simulink model "amk_real_model"  (R2022b)
settings: Solver=FixedStepAuto  StartTime=0.0  StopTime=0.5  FixedStep=1e-6  RelTol=1e-3
values from neighbouring files (symbols this model uses):
  a_fw = log(9)/trfw    [amk_sim.m]    (also in amk_sim_2.m)
  ac = log(9)/tr    [amk_sim.m]    (also in amk_sim_2.m)
  as = log(9)/trs    [amk_sim.m]    (also in amk_sim_2.m)
  ba = 2*k^2*(as*J - 0)/(np^2*psi)    [amk_sim.m]    (also in amk_sim_2.m = 2*k^2*(as*J - bm)/(np^2*psi))
  bm = 0.02    [amk_sim.m]    (also in amk_sim_2.m = 0.008)
  fsw = 8e3    (= 8000)    [amk_sim.m]    (also in amk_sim_2.m)
  I_base = 85.7    [amk_sim.m]    (also in amk_sim_2.m)
  I_max = 85.7    [amk_sim.m]    (also in amk_sim_2.m)
  Icon = 33.5    [amk_sim.m]    (also in amk_sim_2.m)
  Imax_interval = 1.24    [amk_sim.m]    (also in amk_sim_2.m = 5)
  Ipeak = 85.7    [amk_sim.m]    (also in amk_sim_2.m = 87.5)
  J = 2.5*(2.74e-4)    (= 0.000685)    [amk_sim.m]    (also in amk_sim_2.m = 0.000528)
  k = 1    [amk_sim.m]    (also in amk_sim_2.m)
  ki_s = 2*k^2*as^2*J/(np^2*psi)    [amk_sim.m]    (also in amk_sim_2.m)
  kp_s = 2*k^2*as*J/(np^2*psi)    [amk_sim.m]    (also in amk_sim_2.m)
  Ld = Ldm    (= 0.0004)    [amk_sim.m]    (also in amk_sim_2.m = 0.00012)
  Lq = Lqm    (= 0.00052)    [amk_sim.m]    (also in amk_sim_2.m = 0.00024)
  max_temp = 140    [amk_sim.m]    (also in amk_sim_2.m)
  np = 5    [amk_sim.m]    (also in amk_sim_2.m)
  Peak_power = 45000    [amk_sim.m]    (also in amk_sim_2.m = 50000)
  Peak_regen = -15000    [amk_sim.m]    (also in amk_sim_2.m = -1500000)
  psi = 0.047    [amk_sim.m]    (also in amk_sim_2.m = 0.05077789)
  rpm_nom = 20000    [amk_sim.m]    (also in amk_sim_2.m = 12000)
  Rs = 202.5e-3    (= 0.2025)    [amk_sim.m]    (also in amk_sim_2.m)
  sample_time = 1e-4    (= 0.0001)    [amk_sim.m]    (also in amk_sim_2.m = 1e-06)
  temp_threshold = 100    [amk_sim.m]    (also in amk_sim_2.m)
  u_dc = 550    [amk_sim.m]    (also in amk_sim_2.m)
  u_nom = u_dc*k    (= 550)    [amk_sim.m]    (also in amk_sim_2.m)
undefined symbols (not defined in the file or in its folder): Icutoff, rc1, rc2, rc3, rc4, rc5
libraries: spsIGBTDiodeLib x6, simulink x5, spsCurrentMeasurementLib x3, spsSeriesRLCBranchLib x3, spsDCVoltageSourceLib x1, spsPermanentMagnetSynchronousMachineLib x1, dspstat3 x1, spsThreePhaseVIMeasurementLib x1, spsMultimeterLib x1, spsTriangleGeneratorLib x1, sps_lib x1
(part 1 of 4)
settings Model: Creator=alexa  LastModifiedBy=alexa

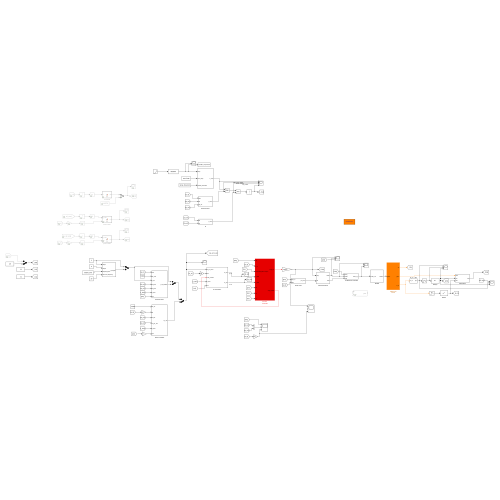
[thumbnail: Simulink's stored preview of the top-level diagram]
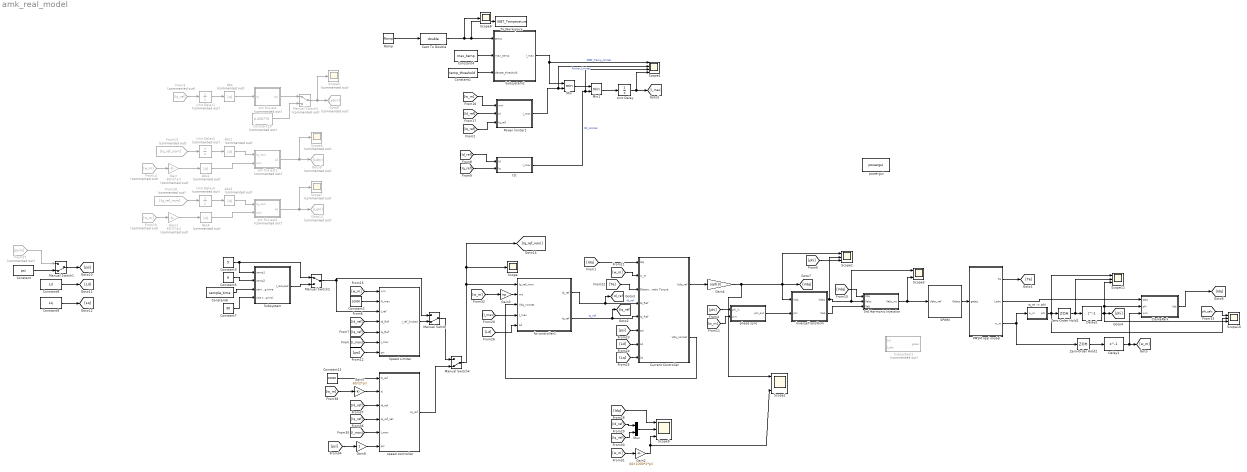
== system amk_real_model ==
  3rd Harmonic Injection : Subsystem
  Abs{,1..4} (5 alike) : Abs  Commented=on  SaturateOnIntegerOverflow=off
  Cast To Double : DataTypeConversion  OutDataTypeStr=double  SaturateOnIntegerOverflow=off  RndMeth=Floor
  ClarkePark : Subsystem
  Constant : Constant  Value=psi
  Constant1 : Constant  Value=temp_threshold
  Constant10 : Constant  Commented=on  Value=0.050779
  Constant11 : Constant  Value=15000
  Constant2 : Constant  Value=10000
  Constant3 : Constant  Value=5
  Constant4 : Constant  Value=max_temp
  Constant5 : Constant  Value=9
  Constant6 : Constant  Value=sample_time
  Constant7 : Constant  Value=30
  Constant8 : Constant  Value=Ld
  Constant9 : Constant  Value=Lq
  Current Controller : Subsystem
  Delay1 : Delay  DelayLength=1  InitialCondition=0  UseCircularBuffer=on
  Delay2 : Delay  DelayLength=1  InitialCondition=0  UseCircularBuffer=on
  From13 : From  Commented=on  GotoTag=Iq_ref_nom
  From14 : From  Commented=on  GotoTag=w_m
  From18 : From  Commented=on  GotoTag=Iq_ref_nom
  From19 : From  Commented=on  GotoTag=w_m
  From27 : From  Commented=on  GotoTag=psim
  From3 : From  Commented=on  GotoTag=Iq_ref
  Gain : Gain  Commented=on  Gain=60/(2*pi)
  Gain1 : Gain  Commented=on  Gain=60/(2*pi)
  Gain2 : Gain  Gain=60/(1000*2*pi)
  Gain3 : Gain  Gain=np
  Gain4 : Gain  Gain=sqrt(3)
  Gain5 : Gain  Gain=60/(2*pi)
  Gain6 : Gain
  Goto13 : Goto  Commented=on  GotoTag=Lqm
  Goto8 : Goto  Commented=on  GotoTag=psim
  Goto9 : Goto  Commented=on  GotoTag=Ldm
  I2t : Subsystem
  InverseTransform : Subsystem
  Manual Switch : ManualSwitch  CurrentSetting=0
  Manual Switch1 : ManualSwitch  CurrentSetting=0
  Manual Switch2 : ManualSwitch
  Manual Switch3 : ManualSwitch  Commented=on
  Manual Switch4 : ManualSwitch  CurrentSetting=0
  Min : MinMax  Inputs=2
  Min1 : MinMax  Inputs=2
  Mux : Mux  Inputs=2
  PMSM real model : Subsystem
  Power limiter1 : Subsystem
  Ramp : simulink/Sources/Ramp  slope=1  start=0  InitialOutput=30
  SPWM : Subsystem
  Scope : Scope
  Scope{1..3,9..11} (6 alike) : Scope  NumInputPorts=3
  Scope4 : Scope  NumInputPorts=4
  Scope5 : Scope  Commented=on
  Scope6 : Scope  Commented=on
  Scope7 : Scope  Commented=on
  Scope8 : Scope
  Speed Limiter : Subsystem
  Subsystem : Subsystem
  Subsystem1 : Subsystem  Commented=on
  Subsystem2 : Subsystem
  To Workspace : ToWorkspace  VariableName=IGBT_Temperature  SampleTime=-1
  Unit Delay : UnitDelay  SampleTime=-1  HasFrameUpgradeWarning=on
  Unit Delay1 : UnitDelay  Commented=on  SampleTime=-1  HasFrameUpgradeWarning=on
  Unit Delay2 : UnitDelay  Commented=on  SampleTime=-1  HasFrameUpgradeWarning=on
  Unit Delay3 : UnitDelay  Commented=on  SampleTime=-1  HasFrameUpgradeWarning=on
  Zero-Order Hold1 : ZeroOrderHold  SampleTime=62e-6
  Zero-Order Hold2 : ZeroOrderHold  SampleTime=62e-6
  fw controller1 : Subsystem
  phase sync : Subsystem
  pm flux est : MATLAB Function  Commented=on  TreatAsAtomicUnit=on
  pm flux est1 : MATLAB Function  Commented=on  TreatAsAtomicUnit=on
  pm flux est2 : MATLAB Function  Commented=on  TreatAsAtomicUnit=on
  powergui : sps_lib/powergui  Priority=1  SimulationMode=Continuous  SampleTime=50e-6  frequency=60  Iterations=50  frequencyindice=0  Pbase=100e6  ErrMax=1e-4  UnitsV=kV  UnitsW=MW  buscounter=0  FunctionMessages=off  echomessages=off  EnableUseOfTLC=off  CurrentSourceSwitches=off  DisableSnubberDevices=off  DisableRonSwitches=off  DisableVfSwitches=off  DisplayEquations=off  AutomaticDiscreteSolvers=off  SolverType=Tustin/Backward Euler (TBE)  Interpol=off  ExternalGateDelay=off  methode=off  Ts=100  x0status=blocks  SPID=on  SwTol=0  HookPort=off  NonlinearTolerance=0  nMaxIteration=15  ContinueOnMaxIteration=off  RestoreLinks=warning  ResistiveCurrentMeasurement=off  Frange=[0:2:500]  Ylog=off  Xlog=on  ShowGrid=off  save=off  variable=ZData  structure=0  ZoomFFT=off  StartTime=0.0  cycles=1  DisplayStyle=1  fundamental=60  FreqAxis=off  MaxFrequency=1000  frequencyindicesteady=1  RmsSteady=1  display=off
  speed controller : Subsystem
  "w_m -> phi" : Subsystem
  wires:
  3rd Harmonic Injection/1(Vabc_inj) -> SPWM/1(Uabc_ref), Scope3/3
  Zero-Order Hold1/1 -> Scope11/2, Delay2/1
  InverseTransform/2(Vab) -> 3rd Harmonic Injection/3(Vab)
  [w_m] -> phase sync/2(wm)
  "w_m -> phi"/1(phi) -> Scope10/2, Scope11/1, Zero-Order Hold1/1
  [phi] -> phase sync/1(phi_in)
  phase sync/1(phi_out) -> InverseTransform/2(phi)
  [Vdq] -> 3rd Harmonic Injection/1(Vdq)
  [phi] -> Scope1/3
  InverseTransform/1(Vabc) -> Scope1/2, Scope3/1, 3rd Harmonic Injection/2(Vabc)
  ClarkePark/1(Idq) -> [Idq]
  PMSM real model/2(I_abc) -> ClarkePark/1(Iabc)
  PMSM real model/3(w_m) -> "w_m -> phi"/1(w_m), Zero-Order Hold2/1
  SPWM/1(Gates) -> PMSM real model/1("gates ")
  PMSM real model/1(Te) -> [Te]
  Current Controller/1("Udq_ref ") -> Gain4/1
  [Iq_ref] -> Mux/2
  From27/1 -> Manual Switch1/1
  [w_m] -> Gain2/1
  From3/1 -> Unit Delay1/1
  Constant10/1 -> Manual Switch3/2
  Abs/1 -> pm flux est/1(Iq)
  Gain/1 -> Abs2/1
  Subsystem/1(I_ramped) -> Manual Switch2/2
  Manual Switch2/1 -> Speed Limiter/3(I_ref), Manual Switch/1
  pm flux est/1(psi) -> Manual Switch3/1
  [Idq] -> Scope9/1
  Abs2/1 -> pm flux est1/2(rpm)
  Constant/1 -> Manual Switch1/2
  [Ld] -> Current Controller/7(Ld)
  pm flux est1/1(Ld) -> Goto9/1, Scope6/1
  Abs1/1 -> pm flux est1/1(Iq_nom)
  Unit Delay2/1 -> Abs1/1
  From13/1 -> Unit Delay2/1
  Constant9/1 -> [Lq]
  [Id_ref] -> Mux/1
  pm flux est2/1(Lq) -> Scope7/1, Goto13/1
  [psi] -> Current Controller/6(psi)
  Gain2/1 -> Scope9/3, Scope2/3
  [Lq] -> Current Controller/8(Lq)
  Manual Switch3/1 -> Scope5/1, Goto8/1
  From14/1 -> Gain/1
  Abs3/1 -> pm flux est2/1(Iq_nom)
  [Id_ref] -> Speed Limiter/4(Id_Ref)
  [Iq_ref] -> Speed Limiter/5(Iq_Ref)
  Mux/1 -> Scope9/2
  From18/1 -> Unit Delay3/1
  Power limiter1/1(I_max) -> Scope4/2, Min/2  "Power_Limiter"
  Constant7/1 -> Subsystem/4(rise time (Amp/ms))
  [psi] -> Speed Limiter/7(psi)
  [Iq_ref] -> Power limiter1/3(Iq_ref)
  [w_m] -> Power limiter1/1(wm)
  Constant1/1 -> Subsystem2/3(derate_threshold)
  Unit Delay/1 -> Scope4/4, [I_max]
  [w_m] -> Gain3/1
  Unit Delay1/1 -> Abs/1
  Gain1/1 -> Abs4/1
  fw controller1/1(Id_ref) -> Current Controller/4(Id_Ref), [Id_ref]  "Id_ref"
  I2t/1(I_max) -> Scope4/3, Min1/2  "I2t_Limiter"
  Abs4/1 -> pm flux est2/2(rpm)
  Subsystem2/1(I_max) -> Min/1, Scope4/1  "IGBT_Temp_limiter"
  Speed Limiter/1(I_ref_limited) -> Manual Switch/2
  [I_max] -> Speed Limiter/6(I_max)
  Unit Delay3/1 -> Abs3/1
  [Iq_ref] -> I2t/2(Iq)
  From19/1 -> Gain1/1
  Constant5/1 -> Subsystem/2(ramp2)
  fw controller1/2(Iq_ref) -> [Iq_ref], Current Controller/5(Iq_Ref)  "Iq_ref"
  [I_max] -> fw controller1/4(I_max)
  Constant4/1 -> Subsystem2/2(max_temp)
  Constant6/1 -> Subsystem/3(sampling time)
  Min/1 -> Min1/1
  [w_m] -> Current Controller/2(w_m)
  [Ld] -> fw controller1/5(Ld)
  [Id_ref] -> I2t/1(Id)
  Constant3/1 -> Subsystem/1(ramp1), Manual Switch2/1
  Current Controller/2(Vdq_nonsat) -> fw controller1/3(Vdq_nonsat)
  Gain3/1 -> fw controller1/2(we)
  [Te] -> Current Controller/3(Electromagnetic Torque)
  Constant2/1 -> Speed Limiter/2(N_max)
  [w_m] -> Speed Limiter/1(wm)
  Cast To Double/1 -> Subsystem2/1(temp), To Workspace/1, Scope8/1
  Min1/1 -> Unit Delay/1
  Ramp/1 -> Cast To Double/1
  [Id_ref] -> Power limiter1/2(Id)
  Manual Switch1/1 -> [psi]
  Constant8/1 -> [Ld]
  [Idq] -> Current Controller/1(Idq)
  Gain4/1 -> Scope2/1, InverseTransform/1(Vdq), Scope1/1, [Vdq]
  Zero-Order Hold2/1 -> Delay1/1
  Delay1/1 -> [w_m], ClarkePark/3(wm)
  Delay2/1 -> Scope11/3, ClarkePark/2(phi), Scope10/3, [phi]
  [phi_calc] -> Scope10/1
  speed controller/1(Iq_ref) -> Manual Switch4/2
  Manual Switch/1 -> Manual Switch4/1
  Manual Switch4/1 -> fw controller1/1(Iq_ref_nom), Scope/1, [Iq_ref_nom]
  [psi] -> Gain6/1
  [I_max] -> speed controller/5(I_max)
  [Iq_ref] -> speed controller/4(Iq_ref_sat)
  [Id_ref] -> speed controller/3(Id_ref)
  Gain5/1 -> speed controller/2(N)
  [w_m] -> Gain5/1
  Constant11/1 -> speed controller/1(N_ref)
  Gain6/1 -> speed controller/6(psi)

== system amk_real_model/3rd Harmonic Injection ==
  note: 3rd harmonic
  Vdq : Inport
  Vabc : Inport  Port=2
  Vab : Inport  Port=3
  Atan2 : Trigonometry  Operator=atan2
  Demux : Demux  Outputs=2
  Demux1 : Demux  Outputs=2
  Gain : Gain  Gain=3
  Gain1 : Gain  Gain=2/sqrt(3)
  Gain2 : Gain  Gain=2/(sqrt(3)*6)
  Product : Product
  Sin : Trigonometry
  Sqrt : Sqrt
  Square : Math  Operator=square
  Square1 : Math  Operator=square
  Sum : Sum  Inputs=|++
  Sum1 : Sum  Inputs=|++
  Vabc_inj : Outport
  wires:
  Vdq/1 -> Demux/1
  Demux/1 -> Square/1
  Demux/2 -> Square1/1
  Square/1 -> Sum/1
  Square1/1 -> Sum/2
  Sum/1 -> Sqrt/1
  Vab/1 -> Demux1/1
  Demux1/1 -> Atan2/1
  Demux1/2 -> Atan2/2
  Atan2/1 -> Gain/1
  Gain/1 -> Sin/1
  Sqrt/1 -> Product/1
  Sin/1 -> Product/2
  Vabc/1 -> Gain1/1
  Product/1 -> Gain2/1
  Gain2/1 -> [mod_3rd]
  Gain1/1 -> Sum1/1
  [mod_3rd] -> Sum1/2
  Sum1/1 -> Vabc_inj/1

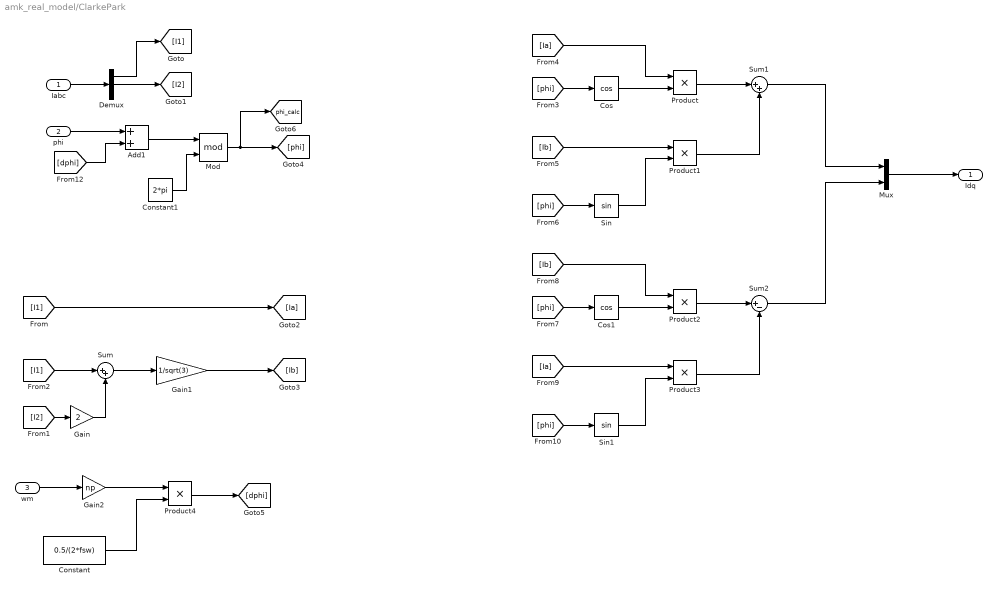
== system amk_real_model/ClarkePark ==
  Iabc : Inport
  phi : Inport  Port=2
  wm : Inport  Port=3
  Add1 : Sum
  Constant : Constant  Value=0.5/(2*fsw)
  Constant1 : Constant  Value=2*pi
  Cos : Trigonometry  Operator=cos
  Cos1 : Trigonometry  Operator=cos
  Demux : Demux  Outputs=3
  Gain : Gain  Gain=2
  Gain1 : Gain  Gain=1/sqrt(3)
  Gain2 : Gain  Gain=np
  Mod : Math  Operator=mod
  Mux : Mux  Inputs=2
  Product{,1..4} (5 alike) : Product
  Sin : Trigonometry
  Sin1 : Trigonometry
  Sum : Sum  Inputs=|++
  Sum1 : Sum  Inputs=|++
  Sum2 : Sum  Inputs=|+-
  Idq : Outport
  tag scope: phi_calc=global
  wires:
  Iabc/1 -> Demux/1
  Demux/1 -> [I1]
  Demux/2 -> [I2]
  [I1] -> [Ia]
  [I1] -> Sum/1
  [I2] -> Gain/1
  Gain/1 -> Sum/2
  Sum/1 -> Gain1/1
  Gain1/1 -> [Ib]
  Cos/1 -> Product/2
  [Ia] -> Product/1
  Product/1 -> Sum1/1
  [phi] -> Sin/1
  [Ib] -> Product1/1
  Sin/1 -> Product1/2
  Product1/1 -> Sum1/2
  Sum1/1 -> Mux/1
  Mux/1 -> Idq/1
  Product3/1 -> Sum2/2
  Sin1/1 -> Product3/2
  [Ia] -> Product3/1
  [phi] -> Sin1/1
  Product2/1 -> Sum2/1
  [Ib] -> Product2/1
  Cos1/1 -> Product2/2
  [phi] -> Cos1/1
  Sum2/1 -> Mux/2
  wm/1 -> Gain2/1
  Gain2/1 -> Product4/1
  Constant/1 -> Product4/2
  Product4/1 -> [dphi]
  [phi] -> Cos/1
  [dphi] -> Add1/2
  phi/1 -> Add1/1
  Add1/1 -> Mod/1
  Mod/1 -> [phi_calc], [phi]
  Constant1/1 -> Mod/2

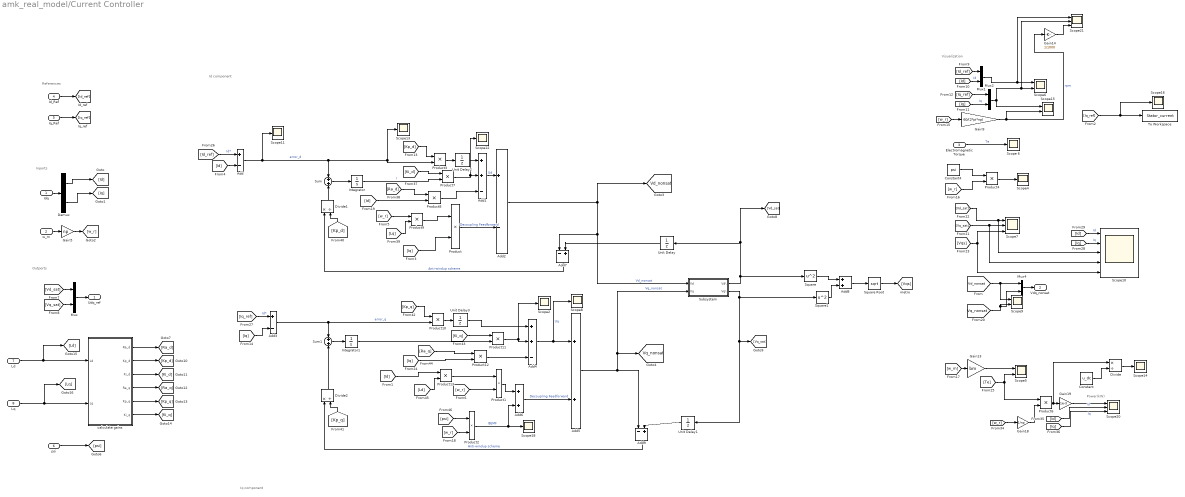
== system amk_real_model/Current Controller ==
  note: References
  note: Id component
  note: Iq component
  note: Inports
  note: Outports
  note: Visualization
  note: Power(kW)
  Idq : Inport
  w_m : Inport  Port=2
  Electromagnetic Torque : Inport  Port=3
  Id_Ref : Inport  Port=4
  Iq_Ref : Inport  Port=5
  psi : Inport  Port=6
  Ld : Inport  Port=7
  Lq : Inport  Port=8
  Add : Sum  Inputs=+-
  Add1 : Sum  Inputs=++-
  Add2 : Sum  Inputs=+-
  Add3 : Sum  Inputs=+-
  Add4 : Sum  Inputs=++-
  Add5 : Sum
  Add6 : Sum
  Add7 : Sum  Inputs=-+
  Add8 : Sum
  Add9 : Sum  Inputs=-+
  Constant : Constant  Value=u_dc
  Constant4 : Constant  Value=psi
  Demux : Demux  Outputs=2
  Divide : Product  Inputs=*/
  Divide1 : Product  Inputs=*/
  Divide2 : Product  Inputs=*/
  Gain13 : Gain  Gain=bm
  Gain14 : Gain  Gain=1/1000
  Gain18 : Gain  Gain=1/np
  Gain19 : Gain  Gain=1e-3
  Gain5 : Gain  Gain=np
  Gain9 : Gain  Gain=60/(2*pi*np)
  Integrator : Integrator
  Integrator1 : Integrator
  Mux{,1..2,4} (4 alike) : Mux  Inputs=2
  Product{,1..4,6..13} (13 alike) : Product
  Scope 6 : Scope
  Scope10 : Scope  NumInputPorts=5
  Scope{2,4,8,11..14,16,18} (9 alike) : Scope
  Scope{5..6,9,15} (4 alike) : Scope  NumInputPorts=2
  Scope20 : Scope  NumInputPorts=3
  Scope21 : Scope  NumInputPorts=3
  Scope7 : Scope  NumInputPorts=3
  Square : Math  Operator=square
  Square Root : Sqrt
  Square1 : Math  Operator=square
  Subsystem : Subsystem
  Sum : Sum
  Sum1 : Sum
  To Workspace : ToWorkspace  VariableName=Stator_current  SampleTime=-1
  Unit Delay{,1..3} (4 alike) : UnitDelay  SampleTime=-1  HasFrameUpgradeWarning=on
  calculate gains : Subsystem
  "Udq_ref " : Outport  VectorParamsAs1DForOutWhenUnconnected=off
  Vdq_nonsat : Outport  Port=2
  tag scope: Vd_nonsat=global, Vq_nonsat=global
  wires:
  Product11/1 -> Add4/2, Scope2/1
  Add4/1 -> Scope8/1, Add5/1  "Uq"
  Add1/1 -> Add2/1  "Ud"
  Product9/1 -> Product/1
  Product10/1 -> Unit Delay3/1
  Sum/1 -> Integrator/1
  Product3/1 -> Unit Delay2/1
  [w_r] -> Product1/2
  Product13/1 -> Product1/1
  Idq/1 -> Demux/1
  Product/1 -> Add2/2  "Decoupling Feedforward"
  Divide1/1 -> Sum/2
  Add2/1 -> [Vd_nonsat], Subsystem/1(Vd), Add7/1  "Vd_nonsat"
  Add7/1 -> Divide1/1  "Anti-windup scheme"
  Sum1/1 -> Integrator1/1
  Add5/1 -> Add9/1, Subsystem/2(Vq), [Vq_nonsat]  "Vq_nonsat"
  Divide2/1 -> Sum1/2
  Add9/1 -> Divide2/1  "Anti-windup scheme"
  Demux/1 -> [Id]
  Demux/2 -> [Iq]
  w_m/1 -> Gain5/1
  Gain5/1 -> [w_r]
  [Vd_sat] -> Mux/1
  [Vq_sat] -> Mux/2
  Mux/1 -> "Udq_ref "/1
  [Id] -> Add/2
  Mux1/1 -> Scope21/1, Scope6/1
  [Id_ref] -> Mux1/1
  [Id] -> Mux1/2  "Id"
  [Iq_ref] -> Mux2/1
  [Iq] -> Mux2/2  "Iq"
  [w_r] -> Gain9/1
  Gain9/1 -> Scope15/2, Gain14/1  "rpm"
  [psi] -> Product2/1
  Product1/1 -> Add6/1
  Add6/1 -> Add5/2  "Decoupling Feedforward"
  Add/1 -> Product3/2, Scope13/1, Sum/1, Scope11/1  "error_d"
  Add3/1 -> Product10/2, Sum1/1  "error_q"
  [Iq] -> Add3/2
  Product7/1 -> Scope12/1, Add1/2
  Square1/1 -> Add8/2
  Square/1 -> Add8/1
  Add8/1 -> Square Root/1
  [Vd_nonsat] -> Scope9/1, Mux4/1
  [Vq_nonsat] -> Mux4/2, Scope9/2
  Square Root/1 -> [Vqs]
  [Vd_sat] -> Scope10/3, Scope7/1
  [Vq_sat] -> Scope10/4, Scope7/2
  [Vqs] -> Scope7/3, Scope10/5
  [w_r] -> Product4/2
  Constant4/1 -> Product4/1
  Product4/1 -> Scope4/1
  Id_Ref/1 -> [Id_ref]
  Iq_Ref/1 -> [Iq_ref]
  Gain13/1 -> Scope5/1
  [Te] -> Product6/1, Scope5/2
  [w_m] -> Gain13/1
  Mux2/1 -> Scope21/2, Scope6/2, Scope15/1
  [Iq] -> Scope10/2  "Iq"
  [Id] -> Scope10/1  "Id"
  [Id_ref] -> Add/1  "Id*"
  Subsystem/1(Vd\) -> Square/1, [Vd_sat], Unit Delay/1
  Subsystem/2(Vq\) -> Square1/1, [Vq_sat], Unit Delay1/1
  [w_r] -> Product2/2
  Product2/1 -> Scope18/1, Add6/2  "BEMF"
  Mux4/1 -> Vdq_nonsat/1
  [Iq_ref] -> Add3/1  "Id*"
  Gain19/1 -> Scope20/1
  [Iq] -> Scope20/3  "Iq"
  [Id] -> Scope20/2  "Id"
  Gain18/1 -> Product6/2
  Product6/1 -> Divide/1, Gain19/1
  [w_r] -> Gain18/1
  Product12/1 -> Add4/3
  Product8/1 -> Add1/3
  Constant/1 -> Divide/2
  Divide/1 -> Scope14/1
  [Id] -> Product8/2
  [Iq] -> Product/2
  [Iq_ref] -> To Workspace/1, Scope16/1
  Electromagnetic Torque/1 -> Scope 6/1  "Te"
  Unit Delay/1 -> Add7/2
  Unit Delay1/1 -> Add9/2
  Gain14/1 -> Scope21/3
  [Kp_d] -> Product3/1
  Integrator/1 -> Product7/2  "I"
  [Ki_d] -> Product7/1
  [Ra_d] -> Product8/1
  [w_r] -> Product9/1
  [Lq] -> Product9/2
  [Kp_d] -> Divide1/2
  [Kp_q] -> Divide2/2
  [Kp_q] -> Product10/1
  [Ki_q] -> Product11/1
  Integrator1/1 -> Product11/2
  [Iq] -> Product12/2
  [Ra_q] -> Product12/1
  [Ld] -> Product13/2
  [Id] -> Product13/1
  Ld/1 -> [Ld], calculate gains/1(Ld)
  Lq/1 -> [Lq], calculate gains/2(Lq)
  psi/1 -> [psi]
  calculate gains/1(Ra_d) -> [Ra_d]
  calculate gains/2(Kp_d) -> [Kp_d]
  calculate gains/3(Ki_d) -> [Ki_d]
  calculate gains/4(Ra_q) -> [Ra_q]
  calculate gains/5(Kp_q) -> [Kp_q]
  calculate gains/6(Ki_q) -> [Ki_q]
  Unit Delay2/1 -> Add1/1
  Unit Delay3/1 -> Add4/1

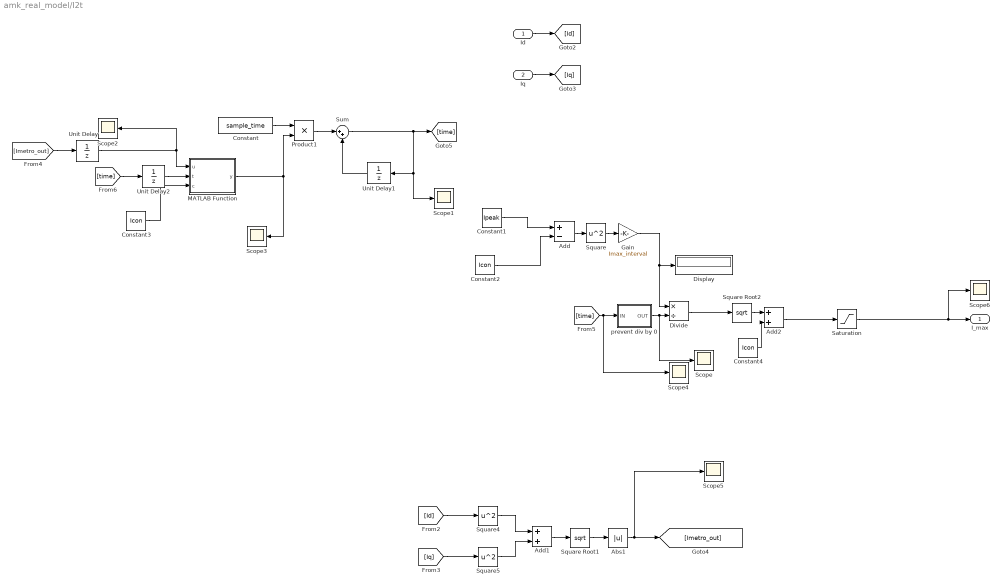
== system amk_real_model/I2t ==
  Id : Inport
  Iq : Inport  Port=2
  Abs1 : Abs  SaturateOnIntegerOverflow=off
  Add : Sum  Inputs=+-
  Add1 : Sum
  Add2 : Sum
  Constant : Constant  Value=sample_time
  Constant1 : Constant  Value=Ipeak
  Constant2 : Constant  Value=Icon
  Constant3 : Constant  Value=Icon
  Constant4 : Constant  Value=Icon
  Display : Display
  Divide : Product  Inputs=*/
  Gain : Gain  Gain=Imax_interval
  MATLAB Function : MATLAB Function  TreatAsAtomicUnit=on
  Product1 : Product
  Saturation : Saturate  UpperLimit=I_max  LowerLimit=0
  Scope{,1..6} (7 alike) : Scope
  Square : Math  Operator=square
  Square Root1 : Sqrt
  Square Root2 : Sqrt
  Square4 : Math  Operator=square
  Square5 : Math  Operator=square
  Sum : Sum  Inputs=|++
  Unit Delay : UnitDelay  SampleTime=-1  HasFrameUpgradeWarning=on
  Unit Delay1 : UnitDelay  SampleTime=-1  HasFrameUpgradeWarning=on
  Unit Delay2 : UnitDelay  SampleTime=-1  HasFrameUpgradeWarning=on
  prevent div by 0 : Subsystem
  I_max : Outport
  wires:
  Iq/1 -> [Iq]
  Id/1 -> [Id]
  Divide/1 -> Square Root2/1
  prevent div by 0/1(OUT) -> Scope/1, Divide/2
  [time] -> Scope4/1, prevent div by 0/1(IN)
  Sum/1 -> Unit Delay1/1, Scope1/1, [time]
  [Imetro_out] -> Unit Delay/1
  [time] -> Unit Delay2/1
  Unit Delay1/1 -> Sum/2
  Add1/1 -> Square Root1/1
  Square5/1 -> Add1/2
  Square4/1 -> Add1/1
  Square Root1/1 -> Abs1/1
  Constant/1 -> Product1/1
  Product1/1 -> Sum/1
  MATLAB Function/1(y) -> Product1/2, Scope3/1
  Constant3/1 -> MATLAB Function/3(c)
  Abs1/1 -> Scope5/1, [Imetro_out]
  Saturation/1 -> I_max/1, Scope6/1
  Unit Delay/1 -> MATLAB Function/1(u), Scope2/1
  Unit Delay2/1 -> MATLAB Function/2(t)
  Gain/1 -> Display/1, Divide/1
  Constant1/1 -> Add/1
  Add/1 -> Square/1
  Constant2/1 -> Add/2
  Square Root2/1 -> Add2/1
  Add2/1 -> Saturation/1
  Constant4/1 -> Add2/2
  Square/1 -> Gain/1
  [Id] -> Square4/1
  [Iq] -> Square5/1

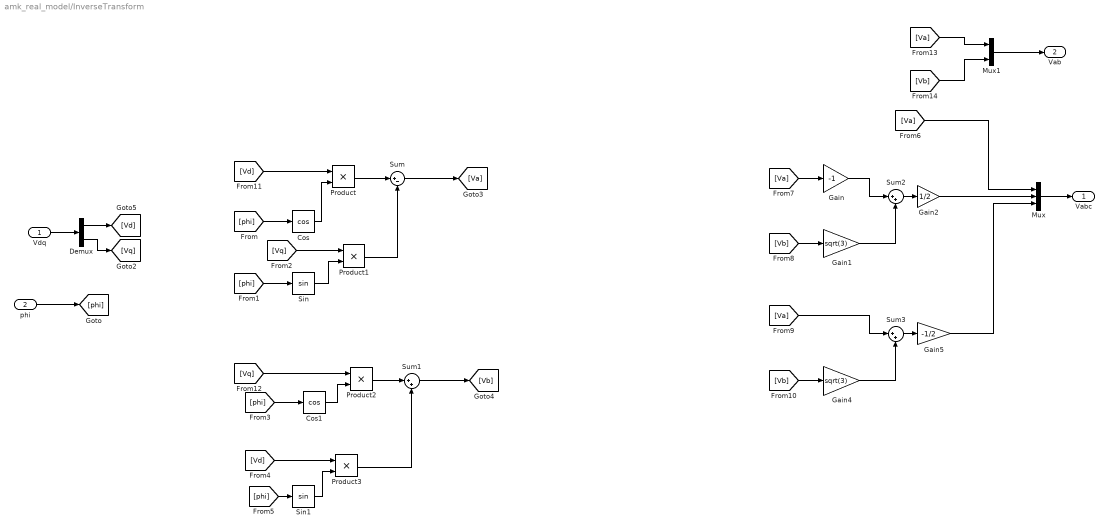
== system amk_real_model/InverseTransform ==
  Vdq : Inport
  phi : Inport  Port=2
  Cos : Trigonometry  Operator=cos
  Cos1 : Trigonometry  Operator=cos
  Demux : Demux  Outputs=2
  Gain : Gain  Gain=-1
  Gain1 : Gain  Gain=sqrt(3)
  Gain2 : Gain  Gain=1/2
  Gain4 : Gain  Gain=sqrt(3)
  Gain5 : Gain  Gain=-1/2
  Mux : Mux  Inputs=3
  Mux1 : Mux  Inputs=2
  Product{,1..3} (4 alike) : Product
  Sin : Trigonometry
  Sin1 : Trigonometry
  Sum : Sum  Inputs=|+-
  Sum1 : Sum  Inputs=|++
  Sum2 : Sum  Inputs=|++
  Sum3 : Sum  Inputs=|++
  Vabc : Outport
  Vab : Outport  Port=2
  wires:
  phi/1 -> [phi]
  [phi] -> Cos/1
  Cos/1 -> Product/2
  Product/1 -> Sum/1
  [phi] -> Sin/1
  [Vq] -> Product1/1
  Sin/1 -> Product1/2
  Product1/1 -> Sum/2
  Cos1/1 -> Product2/2
  [phi] -> Cos1/1
  Product2/1 -> Sum1/1
  Sin1/1 -> Product3/2
  [phi] -> Sin1/1
  [Vd] -> Product3/1
  Product3/1 -> Sum1/2
  Sum/1 -> [Va]
  Sum1/1 -> [Vb]
  [Va] -> Mux/1
  [Va] -> Gain/1
  [Vb] -> Gain1/1
  Gain/1 -> Sum2/1
  Gain1/1 -> Sum2/2
  Sum2/1 -> Gain2/1
  Gain2/1 -> Mux/2
  Sum3/1 -> Gain5/1
  Gain4/1 -> Sum3/2
  [Va] -> Sum3/1
  [Vb] -> Gain4/1
  Vdq/1 -> Demux/1
  Demux/1 -> [Vd]
  Demux/2 -> [Vq]
  [Vd] -> Product/1
  [Vq] -> Product2/1
  Gain5/1 -> Mux/3
  Mux/1 -> Vabc/1
  Mux1/1 -> Vab/1
  [Va] -> Mux1/1
  [Vb] -> Mux1/2

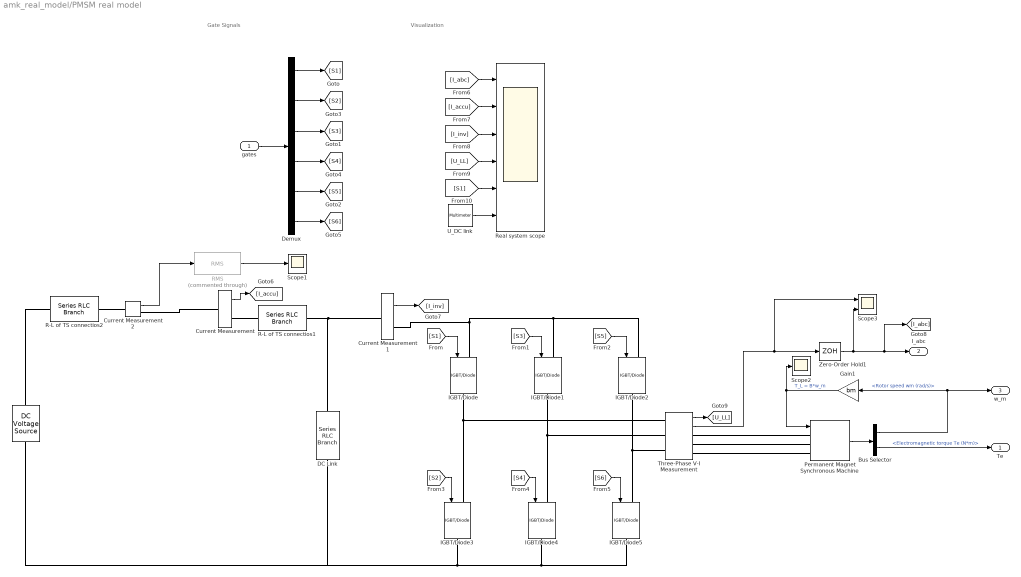
== system amk_real_model/PMSM real model ==
  note: Gate Signals
  note: Visualization
  "gates " : Inport
  " " : spsDCVoltageSourceLib/DC Voltage Source  Description=source block  Amplitude=u_dc  Measurements=None
      settings: AttributesFormatString=\n
  Bus Selector : BusSelector  OutputSignals=Rotor speed wm (rad/s),Electromagnetic torque Te (N*m)
  Current Measurement : spsCurrentMeasurementLib/Current Measurement  PhasorSimulation=off  OutputType=Complex  PSBequivalent=0
  Current Measurement1 : spsCurrentMeasurementLib/Current Measurement  PhasorSimulation=off  OutputType=Complex  PSBequivalent=0
  Current Measurement2 : spsCurrentMeasurementLib/Current Measurement  PhasorSimulation=off  OutputType=Complex  PSBequivalent=0
  DC Link : spsSeriesRLCBranchLib/Series RLC Branch  LConnTagsString=__new0  RConnTagsString=__new0  BranchType=C  Resistance=1  Inductance=1e-3  SetiL0=off  InitialCurrent=0  Capacitance=700e-6  Setx0=off  InitialVoltage=0  Measurements=Branch voltage
  Demux : Demux  Outputs=6
  Gain1 : Gain  Gain=bm
  IGBT/Diode{,1..5} (6 alike) : spsIGBTDiodeLib/IGBT//Diode  Ron=1e-3  Rs=1e5  Cs=inf  Measurements=off
  Permanent Magnet Synchronous Machine : spsPermanentMagnetSynchronousMachineLib/Permanent Magnet Synchronous Machine  NbPhases=3  FluxDistribution=Sinusoidal  RotorType=Salient-pole  MechanicalLoad=Torque Tm  PresetModel=No  ShowDetailedParameters=on  MeasurementBus=off  Resistance=Rs  Inductance=8.5e-3  dqInductances=[Ld Lq]  La=0.00153  MachineConstant=Flux linkage established by magnets (V.s)  Flux=psi  VoltageCst=46.0505  TorqueCst=0.38083  Flat=120  Mechanical=[J 0 np 0]  PolePairs=4  InitialConditions=[0,0, 0,0]  InitialConditions5ph=[0 0 0 0 0 0]  RefAngle=Aligned with phase A axis (original Park)  IterativeDiscreteModel=Trapezoidal non iterative  TsBlock=-1  TsPowergui=0
  R-L of TS connectios1 : spsSeriesRLCBranchLib/Series RLC Branch  LConnTagsString=__new0  RConnTagsString=__new0  BranchType=RL  Resistance=20e-4  Inductance=1e-8  SetiL0=off  InitialCurrent=0  Capacitance=300e-6  Setx0=off  InitialVoltage=0  Measurements=None
  R-L of TS connectios2 : spsSeriesRLCBranchLib/Series RLC Branch  LConnTagsString=__new0  RConnTagsString=__new0  BranchType=RL  Resistance=86.4e-3  Inductance=1e-7  SetiL0=off  InitialCurrent=0  Capacitance=300e-6  Setx0=off  InitialVoltage=0  Measurements=None
  RMS : dspstat3/RMS  Commented=through  run=off  directionMode=Each column  dimension=1  InputProcessing=Columns as channels (frame based)  reset_popup=None
  Real system scope : Scope  NumInputPorts=6
  Scope1 : Scope
  Scope2 : Scope
  Scope3 : Scope  NumInputPorts=2
  Three-Phase V-I Measurement : spsThreePhaseVIMeasurementLib/Three-Phase V-I Measurement  VoltageMeasurement=phase-to-phase  SetLabelV=off  LabelV=Vabc  Vpu=off  VpuLL=off  CurrentMeasurement=yes  SetLabelI=off  LabelI=Iabc  Ipu=off  Pbase=100e6  Vbase=500e3  OutputType=Complex  PhasorSimulation=off  PSBequivalent=0
  U_DC link : spsMultimeterLib/Multimeter  L=1  sel=1  yselected={}  Gain=1  OutputType=Complex  PlotAtSimulationStop=off  PhasorSimulation=off
  Zero-Order Hold1 : ZeroOrderHold  SampleTime=62e-6
  Te : Outport  VectorParamsAs1DForOutWhenUnconnected=off
  I_abc : Outport  Port=2  VectorParamsAs1DForOutWhenUnconnected=off
  w_m : Outport  Port=3  VectorParamsAs1DForOutWhenUnconnected=off
  wires:
  [S2] -> IGBT/Diode3/1
  [S3] -> IGBT/Diode1/1
  Gain1/1 -> Permanent Magnet Synchronous Machine/1, Scope2/1  "T_L = B*w_m"
  [S1] -> IGBT/Diode/1
  [S6] -> IGBT/Diode5/1
  [S4] -> IGBT/Diode4/1
  [S5] -> IGBT/Diode2/1
  Permanent Magnet Synchronous Machine/1 -> Bus Selector/1
  Bus Selector/1 -> Gain1/1, w_m/1  "<Rotor speed wm (rad/s)>"
  Bus Selector/2 -> Te/1  "<Electromagnetic torque Te (N*m)>"
  "gates "/1 -> Demux/1
  Demux/1 -> [S1]
  Demux/2 -> [S2]
  Demux/3 -> [S3]
  Demux/4 -> [S4]
  Demux/5 -> [S5]
  Demux/6 -> [S6]
  Three-Phase V-I Measurement/2 -> Scope3/1, Zero-Order Hold1/1
  Current Measurement/1 -> [I_accu]
  Current Measurement1/1 -> [I_inv]
  [I_abc] -> Real system scope/1
  [I_accu] -> Real system scope/2
  [I_inv] -> Real system scope/3
  Three-Phase V-I Measurement/1 -> [U_LL]
  [U_LL] -> Real system scope/4
  [S1] -> Real system scope/5
  U_DC link/1 -> Real system scope/6
  Zero-Order Hold1/1 -> Scope3/2, I_abc/1, [I_abc]
  Current Measurement2/1 -> RMS/1
  RMS/1 -> Scope1/1
  connections:
  Three-Phase V-I Measurement/RConn2 -- Permanent Magnet Synchronous Machine/LConn2
  Current Measurement/RConn1 -- R-L of TS connectios1/RConn1
  IGBT/Diode2/RConn1 -- IGBT/Diode5/LConn1 -- Three-Phase V-I Measurement/LConn3
  IGBT/Diode1/RConn1 -- IGBT/Diode4/LConn1 -- Three-Phase V-I Measurement/LConn2
  Three-Phase V-I Measurement/RConn1 -- Permanent Magnet Synchronous Machine/LConn1
  IGBT/Diode/RConn1 -- Three-Phase V-I Measurement/LConn1 -- IGBT/Diode3/LConn1
  IGBT/Diode3/RConn1 -- " "/LConn1 -- DC Link/RConn1 -- IGBT/Diode4/RConn1 -- IGBT/Diode5/RConn1
  Three-Phase V-I Measurement/RConn3 -- Permanent Magnet Synchronous Machine/LConn3
  IGBT/Diode/LConn1 -- IGBT/Diode1/LConn1 -- IGBT/Diode2/LConn1 -- Current Measurement1/RConn1
  R-L of TS connectios1/LConn1 -- Current Measurement1/LConn1 -- DC Link/LConn1
  R-L of TS connectios2/RConn1 -- " "/RConn1
  Current Measurement2/LConn1 -- R-L of TS connectios2/LConn1
  Current Measurement2/RConn1 -- Current Measurement/LConn1

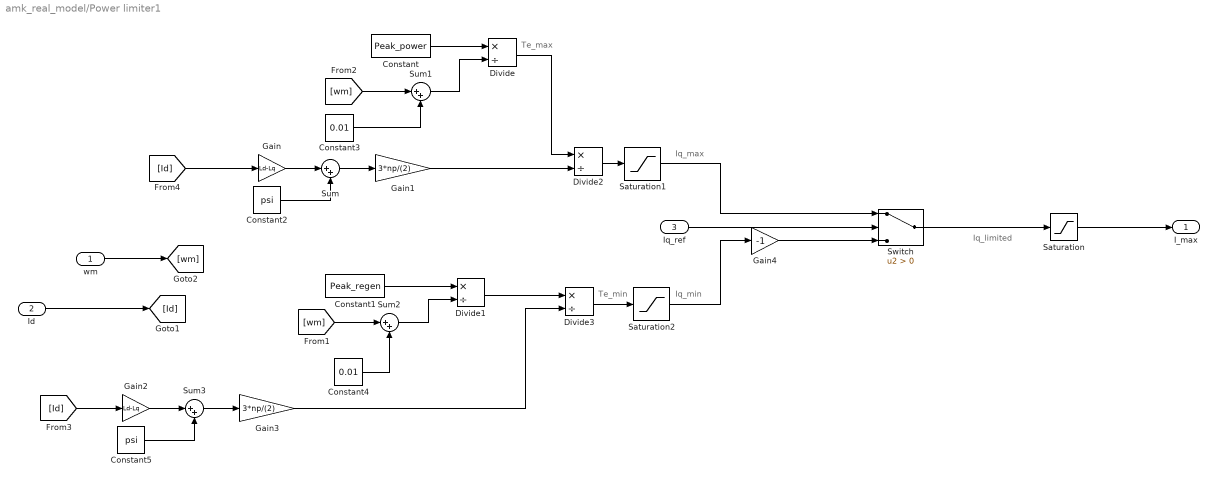
== system amk_real_model/Power limiter1 ==
  note: Te_max
  note: Iq_limited
  note: Iq_max
  note: Iq_min
  note: Te_min
  wm : Inport
  Id : Inport  Port=2
  Iq_ref : Inport  Port=3
  Constant : Constant  Value=Peak_power
  Constant1 : Constant  Value=Peak_regen
  Constant2 : Constant  Value=psi
  Constant3 : Constant  Value=0.01
  Constant4 : Constant  Value=0.01
  Constant5 : Constant  Value=psi
  Divide{,1..3} (4 alike) : Product  Inputs=*/
  Gain : Gain  Gain=Ld-Lq
  Gain1 : Gain  Gain=3*np/(2)
  Gain2 : Gain  Gain=Ld-Lq
  Gain3 : Gain  Gain=3*np/(2)
  Gain4 : Gain  Gain=-1
  Saturation : Saturate  UpperLimit=I_max  LowerLimit=-I_max
  Saturation1 : Saturate  UpperLimit=10000  LowerLimit=-10000
  Saturation2 : Saturate  UpperLimit=10000  LowerLimit=-10000
  Sum{,1..3} (4 alike) : Sum  Inputs=|++
  Switch : Switch  Criteria=u2 > Threshold  SaturateOnIntegerOverflow=off  InputSameDT=off
  I_max : Outport
  wires:
  Sum2/1 -> Divide1/2
  [wm] -> Sum2/1
  Constant4/1 -> Sum2/2
  Saturation2/1 -> Gain4/1
  Saturation1/1 -> Switch/1
  Constant3/1 -> Sum1/2
  [wm] -> Sum1/1
  Sum1/1 -> Divide/2
  Divide2/1 -> Saturation1/1
  Divide3/1 -> Saturation2/1
  Divide/1 -> Divide2/1
  Constant1/1 -> Divide1/1
  Constant/1 -> Divide/1
  Divide1/1 -> Divide3/1
  Switch/1 -> Saturation/1
  wm/1 -> [wm]
  Iq_ref/1 -> Switch/2
  Gain/1 -> Sum/1
  Constant2/1 -> Sum/2
  Sum/1 -> Gain1/1
  Sum3/1 -> Gain3/1
  [Id] -> Gain2/1
  Gain2/1 -> Sum3/1
  Constant5/1 -> Sum3/2
  [Id] -> Gain/1
  Gain3/1 -> Divide3/2
  Gain1/1 -> Divide2/2
  Id/1 -> [Id]
  Gain4/1 -> Switch/3
  Saturation/1 -> I_max/1

== system amk_real_model/SPWM ==
  Uabc_ref : Inport
  Add : Sum  Inputs=+-
  Add1 : Sum  Inputs=+-
  Add2 : Sum  Inputs=+-
  Compare To Zero : simulink/Logic and Bit Operations/Compare To Zero  relop=>=  OutDataTypeStr=boolean  ZeroCross=off
  Compare To Zero1 : simulink/Logic and Bit Operations/Compare To Zero  relop=>=  OutDataTypeStr=boolean  ZeroCross=off
  Compare To Zero2 : simulink/Logic and Bit Operations/Compare To Zero  relop=>=  OutDataTypeStr=boolean  ZeroCross=off
  Delay1 : Delay  DelayLength=1  InitialCondition=0  UseCircularBuffer=on
  Demux : Demux  Outputs=3
  Gain : Gain  Gain=1/u_dc
  Mux : Mux  Inputs=6
  NOT : Logic  Operator=NOT  IconShape=distinctive  AllPortsSameDT=off  OutDataTypeStr=boolean
  NOT1 : Logic  Operator=NOT  IconShape=distinctive  AllPortsSameDT=off  OutDataTypeStr=boolean
  NOT2 : Logic  Operator=NOT  IconShape=distinctive  AllPortsSameDT=off  OutDataTypeStr=boolean
  Scope : Scope  NumInputPorts=2
  Scope1 : Scope  NumInputPorts=3
  Triangle Generator1 : spsTriangleGeneratorLib/Triangle Generator  Freq=fsw  Phase=90  Ts=1e-6
  Zero-Order Hold : ZeroOrderHold  SampleTime=62e-6
  Gates : Outport  VectorParamsAs1DForOutWhenUnconnected=off
  wires:
  Triangle Generator1/1 -> Add/2, Add2/2, Add1/2, Scope/1
  Add/1 -> Compare To Zero/1
  Compare To Zero/1 -> NOT/1, Mux/1
  Add2/1 -> Compare To Zero2/1
  Compare To Zero1/1 -> Mux/3, NOT1/1
  Compare To Zero2/1 -> Mux/5, NOT2/1
  NOT1/1 -> Mux/4
  Demux/1 -> Scope/2, Add/1
  NOT2/1 -> Mux/6
  Gain/1 -> Scope1/1, Delay1/1  "scale for triangle  comparison"
  Add1/1 -> Compare To Zero1/1
  Demux/2 -> Add1/1
  Uabc_ref/1 -> Gain/1
  Demux/3 -> Add2/1
  NOT/1 -> Mux/2
  Mux/1 -> Gates/1
  Zero-Order Hold/1 -> Scope1/3, Demux/1
  Delay1/1 -> Scope1/2, Zero-Order Hold/1

== system amk_real_model/Speed Limiter ==
  note: input
  wm : Inport
  N_max : Inport  Port=2
  I_ref : Inport  Port=3
  Id_Ref : Inport  Port=4
  Iq_Ref : Inport  Port=5
  I_max : Inport  Port=6
  psi : Inport  Port=7
  Constant2 : Constant  Value=0
  Gain4 : Gain  Gain=60/(2*pi)
  Max : MinMax  Function=max  Inputs=2
  Min : MinMax  Inputs=2
  Scope : Scope  NumInputPorts=2
  Sign : Signum
  Switch : Switch  Criteria=u2 > Threshold  SaturateOnIntegerOverflow=off  InputSameDT=off
  speed controller : Subsystem
  speed controller1 : Subsystem
  I_ref_limited : Outport
  wires:
  speed controller1/1(Iq_ref) -> Max/2
  Max/1 -> Switch/3
  I_ref/1 -> Max/1, Sign/1, Scope/2, Min/2
  [Iq_ref] -> speed controller/4(Iq_ref_sat)
  [Id_ref] -> speed controller/3(Id_ref)
  speed controller/1(Iq_ref) -> Scope/1, Min/1
  Gain4/1 -> speed controller1/2(N), speed controller/2(N)
  N_max/1 -> speed controller/1(N_ref)
  Constant2/1 -> speed controller1/1(N_ref)
  Min/1 -> Switch/1
  Sign/1 -> Switch/2
  wm/1 -> Gain4/1
  Switch/1 -> I_ref_limited/1
  Iq_Ref/1 -> [Iq_ref]
  I_max/1 -> [I_max]
  [I_max] -> speed controller1/5(I_max)
  [I_max] -> speed controller/5(I_max)
  [psi] -> speed controller/6(psi)
  [Id_ref] -> speed controller1/3(Id_ref)
  [Iq_ref] -> speed controller1/4(Iq_ref_sat)
  [psi] -> speed controller1/6(psi)
  psi/1 -> [psi]
  Id_Ref/1 -> [Id_ref]

== system amk_real_model/Subsystem ==
  ramp1 : Inport
  ramp2 : Inport  Port=2
  sampling time : Inport  Port=3
  rise time (Amp/ms) : Inport  Port=4
  Constant5 : Constant  Value=0
  Gain : Gain  Gain=1000
  Gain1 : Gain  Gain=0.1
  Max : MinMax  Function=max  Inputs=2
  Memory1 : Memory
  Memory2 : Memory
  Min : MinMax  Inputs=2
  Product : Product
  Product1 : Product
  Step3 : Step  Time=0.25  Before=1  After=-1  SampleTime=0
  Sum1 : Sum  Inputs=|+++
  Sum4 : Sum  Inputs=|-+
  Switch1 : Switch  Criteria=u2 > Threshold  SaturateOnIntegerOverflow=off  InputSameDT=off
  Switch2 : Switch  Criteria=u2 > Threshold  SaturateOnIntegerOverflow=off  InputSameDT=off
  I_ramped : Outport
  wires:
  Sum1/1 -> Memory2/1, Max/1, Sum4/1, Memory1/1
  Switch2/1 -> Product1/2
  Memory2/1 -> Switch2/2
  Product1/1 -> Sum1/1
  Memory1/1 -> Sum1/3
  Gain1/1 -> Switch2/3
  Switch1/1 -> Max/2
  Step3/1 -> Switch1/2, Product1/1  "Id*"
  Sum4/1 -> Sum1/2
  Constant5/1 -> Switch1/1
  Min/1 -> Sum4/2, I_ramped/1
  ramp2/1 -> Switch1/3
  ramp1/1 -> Min/1
  rise time (Amp/ms)/1 -> Gain/1
  sampling time/1 -> Product/2
  Gain/1 -> Product/1
  Product/1 -> Switch2/1, Gain1/1
  Max/1 -> Min/2

== system amk_real_model/Subsystem1 ==
  In1 : Inport
  I_abc : Inport  Port=2
  Constant : Constant  Value=200
  Constant5 : Constant  Value=0
  Demux : Demux  Outputs=3
  Demux1 : Demux  Outputs=3
  Scope : Scope  NumInputPorts=2
  Switch : Switch  Criteria=u2 > Threshold  Threshold=Icutoff  SaturateOnIntegerOverflow=off  InputSameDT=off
  Switch1 : Switch  Criteria=u2 > Threshold  Threshold=Icutoff  SaturateOnIntegerOverflow=off  InputSameDT=off
  Switch2 : Switch  Criteria=u2 > Threshold  Threshold=Icutoff  SaturateOnIntegerOverflow=off  InputSameDT=off
  Transfer Fcn : TransferFcn  Numerator=[rc1]  Denominator=[1 rc1]
  Transfer Fcn1 : TransferFcn  Numerator=[rc2]  Denominator=[1 rc2]
  Transfer Fcn2 : TransferFcn  Numerator=[rc3]  Denominator=[1 rc3]
  Transfer Fcn3 : TransferFcn  Numerator=[rc4]  Denominator=[1 rc4]
  Transfer Fcn4 : TransferFcn  Numerator=[rc5]  Denominator=[1 rc5]
  Transport Delay : TransportDelay  DelayTime=1e-6
  "gates " : Outport
  wires:
  Transfer Fcn/1 -> Transfer Fcn1/1
  I_abc/1 -> Demux/1
  Switch2/1 -> Transfer Fcn/1
  Demux/1 -> Switch2/3
  Constant/1 -> Switch2/1
  Constant5/1 -> Switch/1
  In1/1 -> Switch/3
  Transfer Fcn1/1 -> Transfer Fcn2/1
  Switch/1 -> "gates "/1
  Transport Delay/1 -> Switch2/2, Switch/2
  Transfer Fcn2/1 -> Transfer Fcn3/1
  Transfer Fcn3/1 -> Transfer Fcn4/1
  Transfer Fcn4/1 -> Transport Delay/1

== system amk_real_model/Subsystem2 ==
  temp : Inport
  max_temp : Inport  Port=2
  derate_threshold : Inport  Port=3
  Add : Sum  Inputs=+-
  Add1 : Sum  Inputs=+-
  Add2 : Sum  Inputs=+-
  Constant : Constant  Value=I_max
  Divide : Product  Inputs=*/
  Product : Product
  Saturation : Saturate  UpperLimit=1000  LowerLimit=0
  Scope : Scope  NumInputPorts=2
  Square : Math  Operator=square
  I_max : Outport
  wires:
  max_temp/1 -> Add/1
  Add/1 -> [distance]
  derate_threshold/1 -> [derate_threshold], Add/2
  [derate_threshold] -> Add1/2
  temp/1 -> Add1/1
  Add1/1 -> Saturation/1
  Saturation/1 -> [diff]
  [distance] -> Add2/1
  [diff] -> Add2/2
  Add2/1 -> Divide/1
  [distance] -> Divide/2
  Divide/1 -> Square/1
  Constant/1 -> Product/2, Scope/2
  Square/1 -> Product/1
  Product/1 -> Scope/1, I_max/1

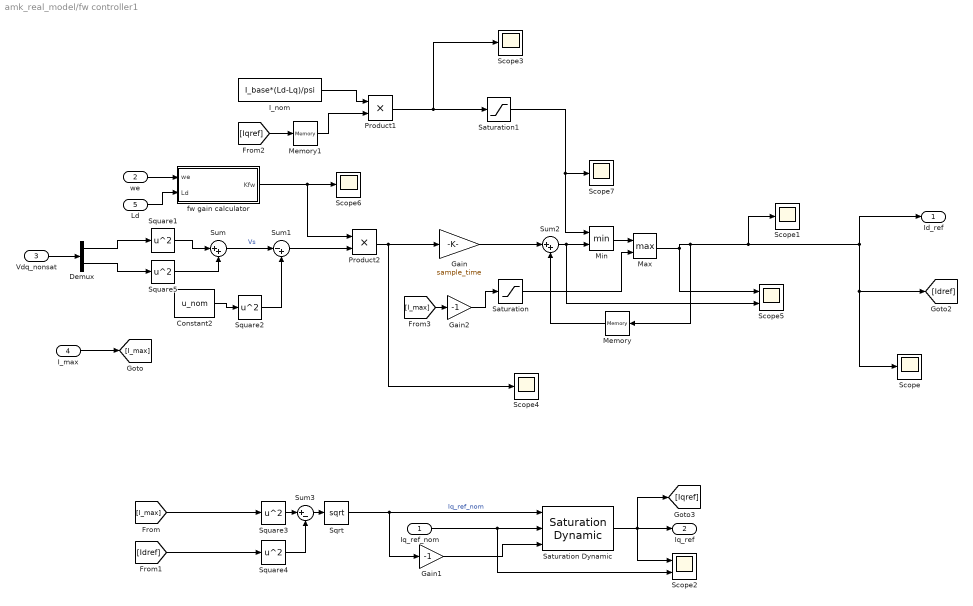
== system amk_real_model/fw controller1 ==
  Iq_ref_nom : Inport
  we : Inport  Port=2
  Vdq_nonsat : Inport  Port=3
  I_max : Inport  Port=4
  Ld : Inport  Port=5
  Constant2 : Constant  Value=u_nom
  Demux : Demux  Outputs=2
  Gain : Gain  Gain=sample_time
  Gain1 : Gain  Gain=-1
  Gain2 : Gain  Gain=-1
  I_nom : Constant  Value=I_base*(Ld-Lq)/psi
  Max : MinMax  Function=max  Inputs=2
  Memory : Memory
  Memory1 : Memory
  Min : MinMax  Inputs=2
  Product1 : Product
  Product2 : Product
  Saturation : Saturate  UpperLimit=-50  LowerLimit=-200
  Saturation Dynamic : simulink/Discontinuities/Saturation Dynamic  OutMin=[]  OutMax=[]  OutDataTypeStr=Inherit: Same as second input  OutDataType=fixdt(1, 16)  OutScaling=2^-10  DoSatur=off
  Saturation1 : Saturate  UpperLimit=20  LowerLimit=-20
  Scope{,1,3..4,6..7} (6 alike) : Scope
  Scope2 : Scope  NumInputPorts=2
  Scope5 : Scope  NumInputPorts=2
  Sqrt : Sqrt
  Square{1..5} (5 alike) : Math  Operator=square
  Sum : Sum  Inputs=|++
  Sum1 : Sum  Inputs=|-+
  Sum2 : Sum  Inputs=|++
  Sum3 : Sum  Inputs=|+-
  fw gain calculator : Subsystem
  Id_ref : Outport
  Iq_ref : Outport  Port=2
  wires:
  Max/1 -> Scope5/1, Memory/1, Scope1/1, [Idref], Scope/1, Id_ref/1
  Product2/1 -> Scope4/1, Gain/1
  Sum1/1 -> Product2/2
  fw gain calculator/1(Kfw) -> Scope6/1, Product2/1
  [Iqref] -> Memory1/1
  Square5/1 -> Sum/2
  Square1/1 -> Sum/1
  Vdq_nonsat/1 -> Demux/1
  Demux/1 -> Square1/1
  Demux/2 -> Square5/1
  I_nom/1 -> Product1/1
  Gain1/1 -> Saturation Dynamic/3
  Sum3/1 -> Sqrt/1
  Constant2/1 -> Square2/1
  Sum/1 -> Sum1/1  "Vs"
  Square2/1 -> Sum1/2
  we/1 -> fw gain calculator/1(we)
  Square3/1 -> Sum3/1
  Square4/1 -> Sum3/2
  Sqrt/1 -> Saturation Dynamic/1, Gain1/1  "Iq_ref_nom"
  Saturation Dynamic/1 -> Scope2/1, Iq_ref/1, [Iqref]
  Gain/1 -> Sum2/1
  Sum2/1 -> Min/2, Scope5/2
  Memory/1 -> Sum2/2
  Product1/1 -> Saturation1/1, Scope3/1
  Gain2/1 -> Saturation/1
  Min/1 -> Max/1
  Saturation/1 -> Max/2
  Saturation1/1 -> Min/1, Scope7/1
  Memory1/1 -> Product1/2
  I_max/1 -> [I_max]
  [I_max] -> Gain2/1
  [I_max] -> Square3/1
  Iq_ref_nom/1 -> Scope2/2, Saturation Dynamic/2
  [Idref] -> Square4/1
  Ld/1 -> fw gain calculator/2(Ld)

== system amk_real_model/phase sync ==
  phi_in : Inport
  wm : Inport  Port=2
  Gain : Gain  Gain=2.5*np/(2*fsw)
  Sum : Sum  Inputs=|++
  phi_out : Outport
  wires:
  wm/1 -> Gain/1
  phi_in/1 -> Sum/1
  Sum/1 -> phi_out/1
  Gain/1 -> Sum/2

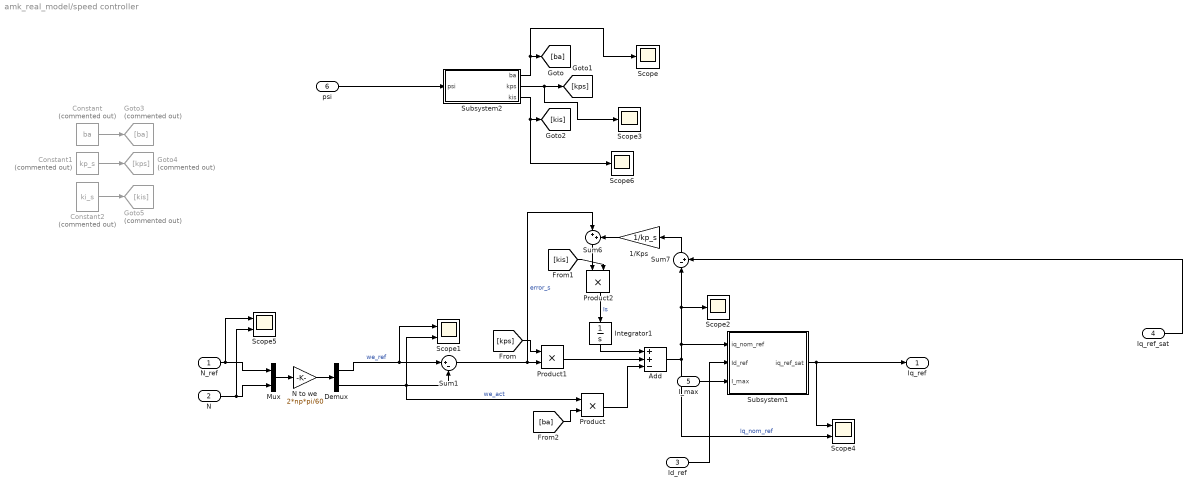
== system amk_real_model/speed controller ==
  N_ref : Inport
  N : Inport  Port=2
  Id_ref : Inport  Port=3
  Iq_ref_sat : Inport  Port=4
  I_max : Inport  Port=5
  psi : Inport  Port=6
  1/Kps : Gain  Gain=1/kp_s
  Add : Sum  Inputs=++-
  Constant : Constant  Commented=on  Value=ba
  Constant1 : Constant  Commented=on  Value=kp_s
  Constant2 : Constant  Commented=on  Value=ki_s
  Demux : Demux  Outputs=2
  Goto3 : Goto  Commented=on  GotoTag=ba
  Goto4 : Goto  Commented=on  GotoTag=kps
  Goto5 : Goto  Commented=on  GotoTag=kis
  Integrator1 : Integrator
  Mux : Mux  Inputs=2
  N to we : Gain  Gain=2*np*pi/60
  Product : Product
  Product1 : Product
  Product2 : Product
  Scope{,2..3,6} (4 alike) : Scope
  Scope1 : Scope  NumInputPorts=2
  Scope4 : Scope  NumInputPorts=2
  Scope5 : Scope  NumInputPorts=2
  Subsystem1 : Subsystem
  Subsystem2 : Subsystem
  Sum1 : Sum  Inputs=|+-
  Sum6 : Sum  Inputs=|++
  Sum7 : Sum  Inputs=|-+
  Iq_ref : Outport
  wires:
  Sum7/1 -> 1/Kps/1
  Add/1 -> Scope2/1, Sum7/1, Subsystem1/1(iq_nom_ref), Scope4/2  "Iq_nom_ref"
  Product1/1 -> Add/2
  1/Kps/1 -> Sum6/2
  Sum1/1 -> Product1/2, Sum6/1  "error_s"
  N_ref/1 -> Scope5/1, Mux/1
  N/1 -> Scope5/2, Mux/2
  [ba] -> Product/2
  Product2/1 -> Integrator1/1  "Is"
  Product/1 -> Add/3
  Demux/1 -> Scope1/1, Sum1/1  "we_ref"
  Demux/2 -> Product/1, Sum1/2, Scope1/2  "we_act"
  Sum6/1 -> Product2/1
  Subsystem1/1(iq_ref_sat) -> Scope4/1, Iq_ref/1
  Mux/1 -> N to we/1
  N to we/1 -> Demux/1
  Integrator1/1 -> Add/1
  Id_ref/1 -> Subsystem1/2(Id_ref)
  I_max/1 -> Subsystem1/3(I_max)
  psi/1 -> Subsystem2/1(psi)
  Subsystem2/1(ba) -> Scope/1, [ba]
  Subsystem2/2(kps) -> Scope3/1, [kps]
  Subsystem2/3(kis) -> Scope6/1, [kis]
  [kps] -> Product1/1
  [kis] -> Product2/2
  Constant/1 -> Goto3/1
  Constant1/1 -> Goto4/1
  Constant2/1 -> Goto5/1
  Iq_ref_sat/1 -> Sum7/2

== system amk_real_model/w_m -> phi ==
  w_m : Inport
  Constant3 : Constant  Value=2*pi
  Gain1 : Gain  Gain=np
  Integrator2 : Integrator
  Mod : Math  Operator=mod  SignedPower=on
  phi : Outport  VectorParamsAs1DForOutWhenUnconnected=off
  wires:
  Constant3/1 -> Mod/2
  Gain1/1 -> Integrator2/1
  Integrator2/1 -> Mod/1
  Mod/1 -> phi/1  "theta rotor"
  w_m/1 -> Gain1/1

== system amk_real_model/Current Controller/Subsystem ==
  Vd : Inport
  Vq : Inport  Port=2
  Constant : Constant  Value=u_nom/(sqrt(3))
  Constant1 : Constant  Value=u_nom/(sqrt(3))
  Divide : Product  Inputs=*/
  Divide1 : Product  Inputs=*/
  Max : MinMax  Function=max  Inputs=2
  Max1 : MinMax  Function=max  Inputs=2
  Product : Product
  Product1 : Product
  Scope : Scope
  Square{,1..3} (4 alike) : Math  Operator=square
  Square Root : Sqrt
  Square Root1 : Sqrt
  Sum : Sum  Inputs=|++
  Sum1 : Sum  Inputs=|++
  Vd\ : Outport
  Vq\ : Outport  Port=2
  wires:
  Square1/1 -> Sum/1
  Square/1 -> Sum/2
  Sum/1 -> Square Root/1
  Square Root/1 -> Max/1
  Constant/1 -> Product/2, Max/2
  Max/1 -> Divide/2
  Divide/1 -> Scope/1, Product/1
  Product/1 -> Vd\/1
  Square3/1 -> Sum1/1
  Constant1/1 -> Product1/2, Max1/2
  Square2/1 -> Sum1/2
  Divide1/1 -> Product1/1
  Vd/1 -> Square2/1, Divide/1, Square1/1
  Vq/1 -> Divide1/1, Square3/1, Square/1
  Square Root1/1 -> Max1/1
  Max1/1 -> Divide1/2
  Sum1/1 -> Square Root1/1
  Product1/1 -> Vq\/1

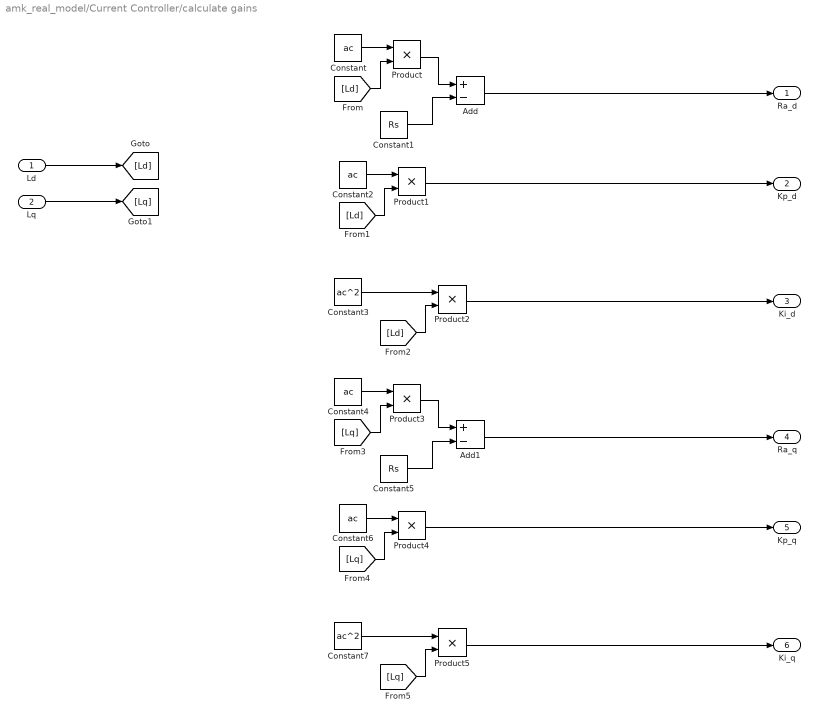
== system amk_real_model/Current Controller/calculate gains ==
  Ld : Inport
  Lq : Inport  Port=2
  Add : Sum  Inputs=+-
  Add1 : Sum  Inputs=+-
  Constant{,2,4,6} (4 alike) : Constant  Value=ac
  Constant1 : Constant  Value=Rs
  Constant3 : Constant  Value=ac^2
  Constant5 : Constant  Value=Rs
  Constant7 : Constant  Value=ac^2
  Product{,1..5} (6 alike) : Product
  Ra_d : Outport
  Kp_d : Outport  Port=2
  Ki_d : Outport  Port=3
  Ra_q : Outport  Port=4
  Kp_q : Outport  Port=5
  Ki_q : Outport  Port=6
  wires:
  Constant/1 -> Product/1
  Ld/1 -> [Ld]
  Lq/1 -> [Lq]
  [Ld] -> Product/2
  Constant1/1 -> Add/2
  Product/1 -> Add/1
  Add/1 -> Ra_d/1
  Product1/1 -> Kp_d/1
  [Ld] -> Product1/2
  Constant2/1 -> Product1/1
  Constant3/1 -> Product2/1
  [Ld] -> Product2/2
  Product2/1 -> Ki_d/1
  Product5/1 -> Ki_q/1
  [Lq] -> Product5/2
  Constant7/1 -> Product5/1
  Constant6/1 -> Product4/1
  [Lq] -> Product4/2
  Product4/1 -> Kp_q/1
  Add1/1 -> Ra_q/1
  Product3/1 -> Add1/1
  Constant5/1 -> Add1/2
  [Lq] -> Product3/2
  Constant4/1 -> Product3/1

== system amk_real_model/I2t/prevent div by 0 ==
  IN : Inport
  Constant : Constant  Value=0.0001
  Switch : Switch  Criteria=u2 > Threshold  Threshold=0.1  SaturateOnIntegerOverflow=off  InputSameDT=off  OutDataTypeStr=Inherit: Same as first input
  OUT : Outport  VectorParamsAs1DForOutWhenUnconnected=off
  wires:
  IN/1 -> Switch/2, Switch/1
  Switch/1 -> OUT/1
  Constant/1 -> Switch/3

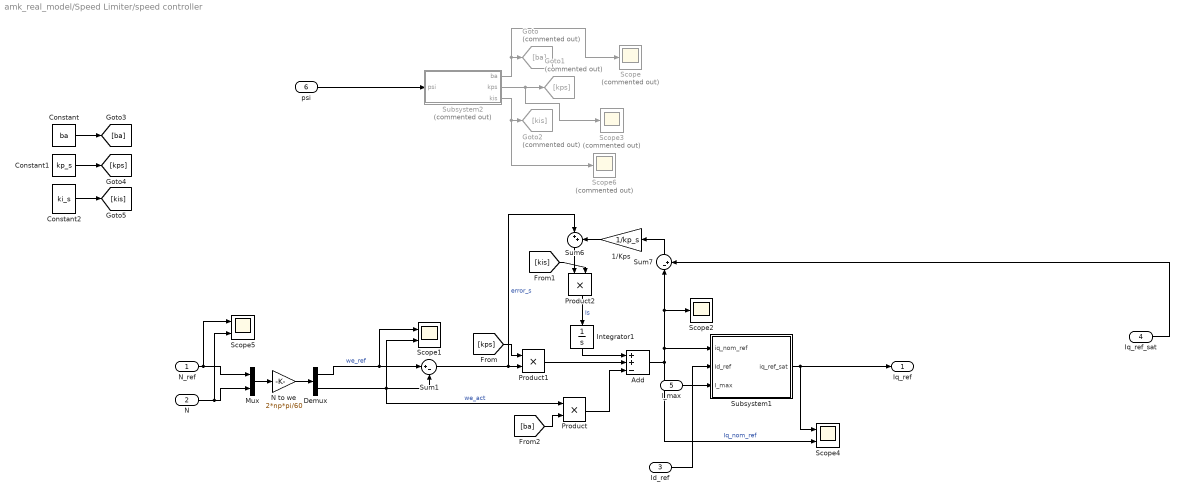
== system amk_real_model/Speed Limiter/speed controller ==
  N_ref : Inport
  N : Inport  Port=2
  Id_ref : Inport  Port=3
  Iq_ref_sat : Inport  Port=4
  I_max : Inport  Port=5
  psi : Inport  Port=6
  1/Kps : Gain  Gain=1/kp_s
  Add : Sum  Inputs=++-
  Constant : Constant  Value=ba
  Constant1 : Constant  Value=kp_s
  Constant2 : Constant  Value=ki_s
  Demux : Demux  Outputs=2
  Goto : Goto  Commented=on  GotoTag=ba
  Goto1 : Goto  Commented=on  GotoTag=kps
  Goto2 : Goto  Commented=on  GotoTag=kis
  Integrator1 : Integrator
  Mux : Mux  Inputs=2
  N to we : Gain  Gain=2*np*pi/60
  Product : Product
  Product1 : Product
  Product2 : Product
  Scope : Scope  Commented=on
  Scope1 : Scope  NumInputPorts=2
  Scope2 : Scope
  Scope3 : Scope  Commented=on
  Scope4 : Scope  NumInputPorts=2
  Scope5 : Scope  NumInputPorts=2
  Scope6 : Scope  Commented=on
  Subsystem1 : Subsystem
  Subsystem2 : Subsystem  Commented=on
  Sum1 : Sum  Inputs=|+-
  Sum6 : Sum  Inputs=|++
  Sum7 : Sum  Inputs=|-+
  Iq_ref : Outport
  wires:
  Sum7/1 -> 1/Kps/1
  Add/1 -> Scope2/1, Sum7/1, Subsystem1/1(iq_nom_ref), Scope4/2  "Iq_nom_ref"
  Product1/1 -> Add/2
  1/Kps/1 -> Sum6/2
  Sum1/1 -> Product1/2, Sum6/1  "error_s"
  N_ref/1 -> Scope5/1, Mux/1
  N/1 -> Scope5/2, Mux/2
  [ba] -> Product/2
  Product2/1 -> Integrator1/1  "Is"
  Product/1 -> Add/3
  Demux/1 -> Scope1/1, Sum1/1  "we_ref"
  Demux/2 -> Product/1, Sum1/2, Scope1/2  "we_act"
  Sum6/1 -> Product2/1
  Subsystem1/1(iq_ref_sat) -> Scope4/1, Iq_ref/1
  Mux/1 -> N to we/1
  N to we/1 -> Demux/1
  Integrator1/1 -> Add/1
  Id_ref/1 -> Subsystem1/2(Id_ref)
  Iq_ref_sat/1 -> Sum7/2
  I_max/1 -> Subsystem1/3(I_max)
  psi/1 -> Subsystem2/1(psi)
  Subsystem2/1(ba) -> Scope/1, Goto/1
  Subsystem2/2(kps) -> Scope3/1, Goto1/1
  Subsystem2/3(kis) -> Scope6/1, Goto2/1
  [kps] -> Product1/1
  [kis] -> Product2/2
  Constant/1 -> [ba]
  Constant1/1 -> [kps]
  Constant2/1 -> [kis]

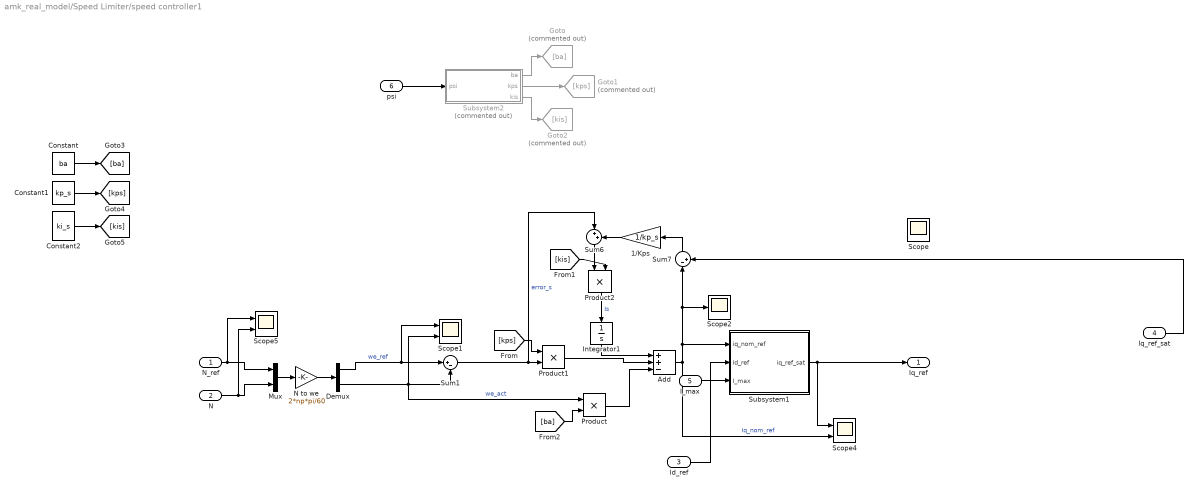
== system amk_real_model/Speed Limiter/speed controller1 ==
  N_ref : Inport
  N : Inport  Port=2
  Id_ref : Inport  Port=3
  Iq_ref_sat : Inport  Port=4
  I_max : Inport  Port=5
  psi : Inport  Port=6
  1/Kps : Gain  Gain=1/kp_s
  Add : Sum  Inputs=++-
  Constant : Constant  Value=ba
  Constant1 : Constant  Value=kp_s
  Constant2 : Constant  Value=ki_s
  Demux : Demux  Outputs=2
  Goto : Goto  Commented=on  GotoTag=ba
  Goto1 : Goto  Commented=on  GotoTag=kps
  Goto2 : Goto  Commented=on  GotoTag=kis
  Integrator1 : Integrator
  Mux : Mux  Inputs=2
  N to we : Gain  Gain=2*np*pi/60
  Product : Product
  Product1 : Product
  Product2 : Product
  Scope : Scope
  Scope1 : Scope  NumInputPorts=2
  Scope2 : Scope
  Scope4 : Scope  NumInputPorts=2
  Scope5 : Scope  NumInputPorts=2
  Subsystem1 : Subsystem
  Subsystem2 : Subsystem  Commented=on
  Sum1 : Sum  Inputs=|+-
  Sum6 : Sum  Inputs=|++
  Sum7 : Sum  Inputs=|-+
  Iq_ref : Outport
  wires:
  [kis] -> Product2/2
  [kps] -> Product1/1
  Subsystem2/3(kis) -> Goto2/1
  Subsystem2/2(kps) -> Goto1/1
  Subsystem2/1(ba) -> Goto/1
  psi/1 -> Subsystem2/1(psi)
  I_max/1 -> Subsystem1/3(I_max)
  Iq_ref_sat/1 -> Sum7/2
  Id_ref/1 -> Subsystem1/2(Id_ref)
  Integrator1/1 -> Add/1
  N to we/1 -> Demux/1
  Mux/1 -> N to we/1
  Subsystem1/1(iq_ref_sat) -> Iq_ref/1, Scope4/1
  Sum6/1 -> Product2/1
  Demux/2 -> Scope1/2, Sum1/2, Product/1  "we_act"
  Demux/1 -> Sum1/1, Scope1/1  "we_ref"
  Product/1 -> Add/3
  Product2/1 -> Integrator1/1  "Is"
  [ba] -> Product/2
  N/1 -> Mux/2, Scope5/2
  N_ref/1 -> Mux/1, Scope5/1
  Sum1/1 -> Sum6/1, Product1/2  "error_s"
  1/Kps/1 -> Sum6/2
  Product1/1 -> Add/2
  Add/1 -> Scope4/2, Subsystem1/1(iq_nom_ref), Sum7/1, Scope2/1  "Iq_nom_ref"
  Sum7/1 -> 1/Kps/1
  Constant1/1 -> [kps]
  Constant/1 -> [ba]
  Constant2/1 -> [kis]

== system amk_real_model/fw controller1/fw gain calculator ==
  we : Inport
  Ld : Inport  Port=2
  Abs : Abs  SaturateOnIntegerOverflow=off
  Constant : Constant  Value=a_fw
  Constant2 : Constant  Value=u_nom
  Constant3 : Constant  Value=rpm_nom
  Divide : Product  Inputs=*/
  Gain : Gain  Gain=2
  Max : MinMax  Function=max  Inputs=2
  N to we : Gain  Gain=2*np*pi/60
  Product : Product  Inputs=3
  Scope1 : Scope  NumInputPorts=2
  Scope2 : Scope
  Kfw : Outport
  wires:
  Constant3/1 -> N to we/1
  we/1 -> Abs/1
  Abs/1 -> Max/2, Scope1/2  "we"
  Gain/1 -> Product/1
  Constant/1 -> Divide/1
  Max/1 -> Product/3
  Constant2/1 -> Product/2
  Product/1 -> Divide/2
  N to we/1 -> Scope1/1, Max/1  "we_max"
  Divide/1 -> Kfw/1, Scope2/1
  Ld/1 -> Gain/1

== system amk_real_model/speed controller/Subsystem1 ==
  iq_nom_ref : Inport
  Id_ref : Inport  Port=2
  I_max : Inport  Port=3
  Add : Sum  Inputs=+-
  Gain : Gain  Gain=-1
  Max : MinMax  Function=max  Inputs=2
  Min : MinMax  Inputs=2
  Scope : Scope
  Square Root : Sqrt
  Square1 : Math  Operator=square
  Square2 : Math  Operator=square
  Unit Delay : UnitDelay  SampleTime=-1  HasFrameUpgradeWarning=on
  iq_ref_sat : Outport
  wires:
  Square2/1 -> Add/1
  iq_nom_ref/1 -> Min/2
  I_max/1 -> Square2/1
  Square1/1 -> Add/2
  Square Root/1 -> Unit Delay/1
  Add/1 -> Square Root/1
  Max/1 -> iq_ref_sat/1
  Gain/1 -> Max/2
  Id_ref/1 -> Square1/1
  Unit Delay/1 -> Min/1, Gain/1, Scope/1
  Min/1 -> Max/1

== system amk_real_model/speed controller/Subsystem2 ==
  psi : Inport
  Constant : Constant  Value=2*k^2*(as*J)/np^2
  Constant1 : Constant  Value=2*k^2*(as*J)/np^2
  Constant2 : Constant  Value=2*k^2*(as^2*J)/np^2
  Divide : Product  Inputs=*/
  Divide1 : Product  Inputs=*/
  Divide2 : Product  Inputs=*/
  ba : Outport
  kps : Outport  Port=2
  kis : Outport  Port=3
  wires:
  Constant/1 -> Divide/1
  psi/1 -> [psi]
  [psi] -> Divide/2
  [psi] -> Divide1/2
  Constant1/1 -> Divide1/1
  Constant2/1 -> Divide2/1
  [psi] -> Divide2/2
  Divide/1 -> ba/1
  Divide1/1 -> kps/1
  Divide2/1 -> kis/1

== system amk_real_model/Speed Limiter/speed controller/Subsystem1 ==
  iq_nom_ref : Inport
  Id_ref : Inport  Port=2
  I_max : Inport  Port=3
  Add : Sum  Inputs=+-
  Gain : Gain  Gain=-1
  Max : MinMax  Function=max  Inputs=2
  Min : MinMax  Inputs=2
  Scope : Scope
  Square Root : Sqrt
  Square1 : Math  Operator=square
  Square2 : Math  Operator=square
  Unit Delay : UnitDelay  SampleTime=-1  HasFrameUpgradeWarning=on
  iq_ref_sat : Outport
  wires:
  Square2/1 -> Add/1
  iq_nom_ref/1 -> Min/2
  I_max/1 -> Square2/1
  Square1/1 -> Add/2
  Square Root/1 -> Unit Delay/1
  Add/1 -> Square Root/1
  Max/1 -> iq_ref_sat/1
  Gain/1 -> Max/2
  Id_ref/1 -> Square1/1
  Unit Delay/1 -> Min/1, Gain/1, Scope/1
  Min/1 -> Max/1

== system amk_real_model/Speed Limiter/speed controller/Subsystem2 ==
  psi : Inport
  Constant : Constant  Value=2*k^2*(as*J)/np^2
  Constant1 : Constant  Value=2*k^2*(as*J)/np^2
  Constant2 : Constant  Value=2*k^2*(as^2*J)/np^2
  Divide : Product  Inputs=*/
  Divide1 : Product  Inputs=*/
  Divide2 : Product  Inputs=*/
  ba : Outport
  kps : Outport  Port=2
  kis : Outport  Port=3
  wires:
  Constant/1 -> Divide/1
  psi/1 -> [psi]
  [psi] -> Divide/2
  [psi] -> Divide1/2
  Constant1/1 -> Divide1/1
  Constant2/1 -> Divide2/1
  [psi] -> Divide2/2
  Divide/1 -> ba/1
  Divide1/1 -> kps/1
  Divide2/1 -> kis/1

== system amk_real_model/Speed Limiter/speed controller1/Subsystem1 ==
  iq_nom_ref : Inport
  Id_ref : Inport  Port=2
  I_max : Inport  Port=3
  Add : Sum  Inputs=+-
  Gain : Gain  Gain=-1
  Max : MinMax  Function=max  Inputs=2
  Min : MinMax  Inputs=2
  Scope : Scope
  Square Root : Sqrt
  Square1 : Math  Operator=square
  Square2 : Math  Operator=square
  Unit Delay : UnitDelay  SampleTime=-1  HasFrameUpgradeWarning=on
  iq_ref_sat : Outport
  wires:
  Id_ref/1 -> Square1/1
  Gain/1 -> Max/2
  Add/1 -> Square Root/1
  Square Root/1 -> Unit Delay/1
  Square1/1 -> Add/2
  I_max/1 -> Square2/1
  iq_nom_ref/1 -> Min/2
  Square2/1 -> Add/1
  Unit Delay/1 -> Min/1, Scope/1, Gain/1
  Min/1 -> Max/1
  Max/1 -> iq_ref_sat/1
